simulink library "foc_blocks"  (R2020b)
settings: Solver=ode45  StartTime=0.0  StopTime=10.0  RelTol=1e-3  EnableMultiTasking=on
values from neighbouring files (symbols this model uses):
  ClockFrequency = 100    [setup_DF_fixp16_alu_av.m]    (also in setup_sim_DF_fixp16_alu.m; setup_verify_DF_fixp16_alu.m)
  constfractionlengthIn = 10    [setup_DF_fixp16_alu_av.m]    (also in setup_sim_DF_fixp16_alu.m; setup_verify_DF_fixp16_alu.m)
  constwordlengthIn = 16    [setup_DF_fixp16_alu_av.m]    (also in setup_sim_DF_fixp16_alu.m; setup_verify_DF_fixp16_alu.m)
  DSPBASampleTime = FoldingFactor / (ClockFrequency * 1e6)    (= 5e-06)    [setup_DF_fixp16_alu_av.m]    (also in setup_sim_DF_fixp16_alu.m; setup_verify_DF_fixp16_alu.m)
  FoldingFactor = 500    [setup_DF_fixp16_alu_av.m]    (also in setup_sim_DF_fixp16_alu.m; setup_verify_DF_fixp16_alu.m)
undefined symbols (not defined in the file or in its folder): AdvDSPBChannelOutDisplay, dpoly, dspba_ChannelInVis, dspba_ChannelOutVis, dspba_internal_get_channel_ports, evalAionMaskParam, latency, primtype, value, x
libraries: DSPBAPrim x559, AlteraGenericMotorLibrary x20, $bdroot x9, DSPBAUtilities x4, DSPBAControl x4
(part 4 of 6)

== system foc_blocks/FL_float_filt/FP_CP1_DSPBA1 ==
  note: Park & Clarke Transform
  I_uw : Inport
  cos_phi_el : Inport  Port=2
  sin_phi_el : Inport  Port=3
  Add : DSPBAPrim/Add  primtype=add  nInputs=evalAionMaskParam(gcb,'value',1)  nOutputs=1  omode=Inherit via internal rule  otype=sfix(16)  scale=2^-15  rndmethod=Unbiased  factor=1  satmethod=Symmetric  shift_vec=[0 1 2 -1]  value=2  inPortNames=[' '; ' ';]  outPortNames=[' ']  dspbaimage=dspba_prim.jpg  text=fprintf('+');  style=Optimised  visibilities=1032  genFPC=off  floatRounding=faithful  advOptions=[]  version=20130821
  Add1 : DSPBAPrim/Add  primtype=add  nInputs=evalAionMaskParam(gcb,'value',1)  nOutputs=1  omode=Inherit via internal rule with word growth  otype=sfix(16)  scale=2^-15  rndmethod=Unbiased  factor=1  satmethod=Symmetric  shift_vec=[0 1 2 -1]  value=2  inPortNames=[' '; ' ';]  outPortNames=[' ']  dspbaimage=dspba_prim.jpg  text=fprintf('+');  style=Optimised  visibilities=1032  genFPC=off  floatRounding=faithful  advOptions=[]  version=20130821
  Altera DSP Builder Advanced : AlteraGenericMotorLibrary/FP_Cur_Ctrl_DSPBA/Altera DSP Builder Advanced  SystemSampleTime=-1  VariantActivationTime=update diagram  Latency=0  AutoFrameSizeCalculation=off
  Demux1 : Demux  Outputs=2
  FPGain : Subsystem  mask{constVal=2}
      mask prompts: constVal "Gain"
      mask Display: color('w');fprintf('FP Gain\n%s', num2str(constVal));port_label('input',1,'a');port_label('output',1,'q');
  FPGain1 : Subsystem  mask{constVal=-1/sqrt(3)}
      mask prompts: constVal "Gain"
      mask Display: color('w');fprintf('FP Gain\n%s', num2str(constVal));port_label('input',1,'a');port_label('output',1,'q');
  Mult{,1..3} (4 alike) : DSPBAPrim/Mult  primtype=mult  nInputs=2  nOutputs=1  omode=Inherit via internal rule  otype=sfix(16)  scale=2^-15  rndmethod=Unbiased  factor=1  satmethod=Symmetric  shift_vec=[0 1 2 -1]  value=0  inPortNames=[' '; ' ';]  outPortNames=[' ']  dspbaimage=dspba_prim.jpg  text=fprintf('X');  style=Optimised  visibilities=8  floatPrecision=float32_m23  floatRounding=faithful  advOptions=[]  version=20130115
  Mux1 : Mux  Inputs=2
  Sub1 : DSPBAPrim/Sub  primtype=sub  nInputs=2  nOutputs=1  omode=Inherit via internal rule  otype=sfix(16)  scale=2^-15  rndmethod=Unbiased  factor=1  satmethod=Symmetric  shift_vec=[0 1 2 -1]  value=0  inPortNames=['+'; '-';]  outPortNames=[' ']  dspbaimage=dspba_prim.jpg  text=fprintf('-');  style=Optimised  visibilities=8  floatRounding=faithful  advOptions=[]  version=20130115
  I_dq : Outport
  wires:
  Sub1/1 -> Mux1/2
  Add/1 -> Mux1/1
  Mux1/1 -> I_dq/1
  Mult3/1 -> Sub1/1
  Mult2/1 -> Sub1/2
  Mult1/1 -> Add/2
  Mult/1 -> Add/1
  cos_phi_el/1 -> Mult/2, Mult3/2
  FPGain1/1(Out1) -> Mult1/1, Mult3/1
  Demux1/1 -> Mult/1, Mult2/2, Add1/1
  Demux1/2 -> FPGain/1(In1)
  I_uw/1 -> Demux1/1
  sin_phi_el/1 -> Mult1/2, Mult2/1
  Add1/1 -> FPGain1/1(In1)
  FPGain/1(Out1) -> Add1/2

== system foc_blocks/FL_float_filt/FP_Inv_Park1 ==
  note: Inverse Park Transform
  I_dq : Inport
  cos_phi_el : Inport  Port=2
  sin_phi_el : Inport  Port=3
  Add : DSPBAPrim/Add  primtype=add  nInputs=evalAionMaskParam(gcb,'value',1)  nOutputs=1  omode=Inherit via internal rule  otype=sfix(16)  scale=2^-15  rndmethod=Unbiased  factor=1  satmethod=Symmetric  shift_vec=[0 1 2 -1]  value=2  inPortNames=[' '; ' ';]  outPortNames=[' ']  dspbaimage=dspba_prim.jpg  text=fprintf('+');  style=Optimised  visibilities=1032  genFPC=off  floatRounding=faithful  advOptions=[]  version=20130821
  Altera DSP Builder Advanced : AlteraGenericMotorLibrary/FP_Cur_Ctrl_DSPBA/Altera DSP Builder Advanced  SystemSampleTime=-1  VariantActivationTime=update diagram  Latency=0  AutoFrameSizeCalculation=off
  Demux1 : Demux  Outputs=2
  Mult{1..4} (4 alike) : DSPBAPrim/Mult  primtype=mult  nInputs=2  nOutputs=1  omode=Inherit via internal rule  otype=sfix(16)  scale=2^-15  rndmethod=Unbiased  factor=1  satmethod=Symmetric  shift_vec=[0 1 2 -1]  value=0  inPortNames=[' '; ' ';]  outPortNames=[' ']  dspbaimage=dspba_prim.jpg  text=fprintf('X');  style=Optimised  visibilities=8  floatPrecision=float32_m23  floatRounding=faithful  advOptions=[]  version=20130115
  Mux2 : Mux  Inputs=2
  Sub1 : DSPBAPrim/Sub  primtype=sub  nInputs=2  nOutputs=1  omode=Inherit via internal rule  otype=sfix(16)  scale=2^-15  rndmethod=Unbiased  factor=1  satmethod=Symmetric  shift_vec=[0 1 2 -1]  value=0  inPortNames=['+'; '-';]  outPortNames=[' ']  dspbaimage=dspba_prim.jpg  text=fprintf('-');  style=Optimised  visibilities=8  floatRounding=faithful  advOptions=[]  version=20130115
  I_alpha_beta : Outport
  wires:
  Mult2/1 -> Add/1
  Mult1/1 -> Add/2
  Mult4/1 -> Sub1/1
  Mult3/1 -> Sub1/2
  Demux1/1 -> Mult2/1, Mult4/1  "I_d"
  cos_phi_el/1 -> Mult1/2, Mult4/2
  Demux1/2 -> Mult1/1, Mult3/1  "I_q"
  sin_phi_el/1 -> Mult2/2, Mult3/2
  I_dq/1 -> Demux1/1
  Mux2/1 -> I_alpha_beta/1
  Sub1/1 -> Mux2/1
  Add/1 -> Mux2/2

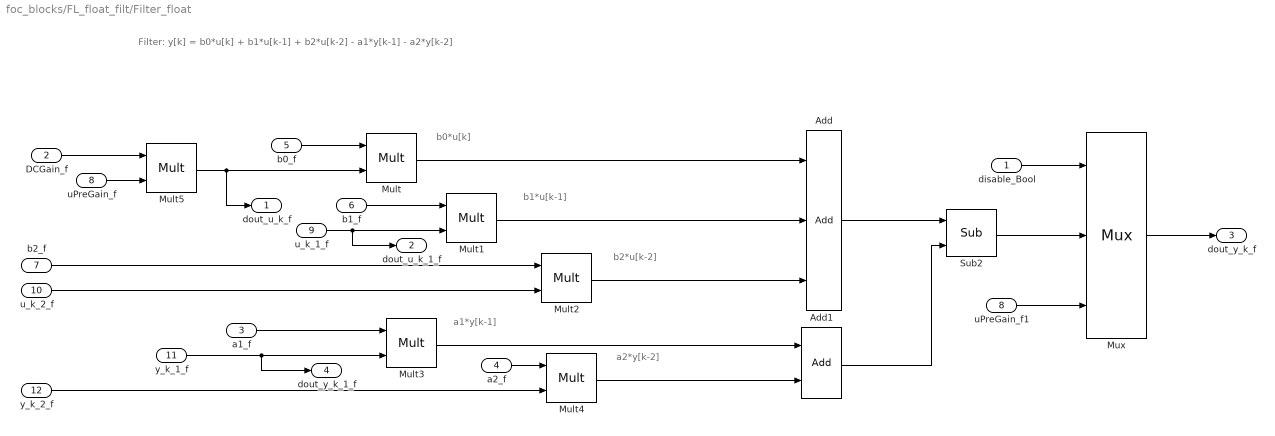
== system foc_blocks/FL_float_filt/Filter_float ==
  note: b0*u[k]
  note: b1*u[k-1]
  note: b2*u[k-2]
  note: a1*y[k-1]
  note: a2*y[k-2]
  note: Filter: y[k] = b0*u[k] + b1*u[k-1] + b2*u[k-2] - a1*y[k-1] - a2*y[k-2]
  disable_Bool : Inport
  DCGain_f : Inport  Port=2
  a1_f : Inport  Port=3
  a2_f : Inport  Port=4
  b0_f : Inport  Port=5
  b1_f : Inport  Port=6
  b2_f : Inport  Port=7
  uPreGain_f : Inport  Port=8
  u_k_1_f : Inport  Port=9
  u_k_2_f : Inport  Port=10
  y_k_1_f : Inport  Port=11
  y_k_2_f : Inport  Port=12
  Add : DSPBAPrim/Add  primtype=add  nInputs=evalAionMaskParam(gcb,'value',1)  nOutputs=1  omode=Inherit via internal rule  otype=sfix(16)  scale=2^-15  rndmethod=Unbiased  factor=1  satmethod=Symmetric  shift_vec=[0 1 2 -1]  value=3  inPortNames=[' '; ' ';]  outPortNames=[' ']  dspbaimage=dspba_prim.jpg  text=fprintf('+');  style=Optimised  visibilities=1032  genFPC=off  floatRounding=faithful  advOptions=[]  version=20130821
  Add1 : DSPBAPrim/Add  primtype=add  nInputs=evalAionMaskParam(gcb,'value',1)  nOutputs=1  omode=Inherit via internal rule  otype=sfix(16)  scale=2^-15  rndmethod=Unbiased  factor=1  satmethod=Symmetric  shift_vec=[0 1 2 -1]  value=2  inPortNames=[' '; ' ';]  outPortNames=[' ']  dspbaimage=dspba_prim.jpg  text=fprintf('+');  style=Optimised  visibilities=1032  genFPC=off  floatRounding=faithful  advOptions=[]  version=20130821
  Mult{,1..5} (6 alike) : DSPBAPrim/Mult  primtype=mult  nInputs=2  nOutputs=1  omode=Inherit via internal rule  otype=sfix(16)  scale=2^-15  rndmethod=Unbiased  factor=1  satmethod=Symmetric  shift_vec=[0 1 2 -1]  value=0  inPortNames=[' '; ' ';]  outPortNames=[' ']  dspbaimage=dspba_prim.jpg  text=fprintf('X');  style=Optimised  visibilities=8  floatPrecision=float32_m23  floatRounding=faithful  advOptions=[]  version=20130115
  Mux : DSPBAPrim/Mux  primtype=mux  nInputs=evalAionMaskParam(gcb,'value',1)+1  nOutputs=1  omode=Inherit via internal rule  otype=sfix(16)  scale=2^-15  rndmethod=Unbiased  factor=1  satmethod=Symmetric  shift_vec=[0 1 2 -1]  value=2  inPortNames=['s'; 'd0'; 'd1'; 'd2'; 'd3'; 'd4'; 'd5'; 'd6'; 'd7'; 'd8'; 'd9';]  outPortNames=[' ']  dspbaimage=dspba_prim.jpg  text=fprintf('%s', primtype);  style=Optimised  visibilities=1032  version=20131025
  Sub2 : DSPBAPrim/Sub  primtype=sub  nInputs=2  nOutputs=1  omode=Inherit via internal rule  otype=sfix(16)  scale=2^-15  rndmethod=Unbiased  factor=1  satmethod=Symmetric  shift_vec=[0 1 2 -1]  value=0  inPortNames=['+'; '-';]  outPortNames=[' ']  dspbaimage=dspba_prim.jpg  text=fprintf('-');  style=Optimised  visibilities=8  floatRounding=faithful  advOptions=[]  version=20130115
  uPreGain_f1 : InportShadow  Port=8
  dout_u_k_f : Outport
  dout_u_k_1_f : Outport  Port=2
  dout_y_k_f : Outport  Port=3
  dout_y_k_1_f : Outport  Port=4
  wires:
  b1_f/1 -> Mult1/1
  y_k_1_f/1 -> dout_y_k_1_f/1, Mult3/2
  u_k_1_f/1 -> dout_u_k_1_f/1, Mult1/2
  Mult4/1 -> Add1/2
  b0_f/1 -> Mult/1
  a1_f/1 -> Mult3/1
  u_k_2_f/1 -> Mult2/2
  b2_f/1 -> Mult2/1
  Mult3/1 -> Add1/1
  Add1/1 -> Sub2/2
  Add/1 -> Sub2/1
  Mult1/1 -> Add/2
  Mult/1 -> Add/1
  a2_f/1 -> Mult4/1
  Mult2/1 -> Add/3
  y_k_2_f/1 -> Mult4/2
  Mult5/1 -> dout_u_k_f/1, Mult/2
  DCGain_f/1 -> Mult5/1
  uPreGain_f/1 -> Mult5/2
  disable_Bool/1 -> Mux/1
  uPreGain_f1/1 -> Mux/3
  Sub2/1 -> Mux/2
  Mux/1 -> dout_y_k_f/1

== system foc_blocks/FL_float_filt/Filter_float1 ==
  note: Filter: y[k] = b0*u[k] + b1*u[k-1] + b2*u[k-2] - a1*y[k-1] - a2*y[k-2]
  note: a2*y[k-2]
  note: a1*y[k-1]
  note: b2*u[k-2]
  note: b1*u[k-1]
  note: b0*u[k]
  disable_Bool : Inport
  DCGain_f : Inport  Port=2
  a1_f : Inport  Port=3
  a2_f : Inport  Port=4
  b0_f : Inport  Port=5
  b1_f : Inport  Port=6
  b2_f : Inport  Port=7
  uPreGain_f : Inport  Port=8
  u_k_1_f : Inport  Port=9
  u_k_2_f : Inport  Port=10
  y_k_1_f : Inport  Port=11
  y_k_2_f : Inport  Port=12
  Add : DSPBAPrim/Add  primtype=add  nInputs=evalAionMaskParam(gcb,'value',1)  nOutputs=1  omode=Inherit via internal rule  otype=sfix(16)  scale=2^-15  rndmethod=Unbiased  factor=1  satmethod=Symmetric  shift_vec=[0 1 2 -1]  value=3  inPortNames=[' '; ' ';]  outPortNames=[' ']  dspbaimage=dspba_prim.jpg  text=fprintf('+');  style=Optimised  visibilities=1032  genFPC=off  floatRounding=faithful  advOptions=[]  version=20130821
  Add1 : DSPBAPrim/Add  primtype=add  nInputs=evalAionMaskParam(gcb,'value',1)  nOutputs=1  omode=Inherit via internal rule  otype=sfix(16)  scale=2^-15  rndmethod=Unbiased  factor=1  satmethod=Symmetric  shift_vec=[0 1 2 -1]  value=2  inPortNames=[' '; ' ';]  outPortNames=[' ']  dspbaimage=dspba_prim.jpg  text=fprintf('+');  style=Optimised  visibilities=1032  genFPC=off  floatRounding=faithful  advOptions=[]  version=20130821
  Mult{,1..5} (6 alike) : DSPBAPrim/Mult  primtype=mult  nInputs=2  nOutputs=1  omode=Inherit via internal rule  otype=sfix(16)  scale=2^-15  rndmethod=Unbiased  factor=1  satmethod=Symmetric  shift_vec=[0 1 2 -1]  value=0  inPortNames=[' '; ' ';]  outPortNames=[' ']  dspbaimage=dspba_prim.jpg  text=fprintf('X');  style=Optimised  visibilities=8  floatPrecision=float32_m23  floatRounding=faithful  advOptions=[]  version=20130115
  Mux : DSPBAPrim/Mux  primtype=mux  nInputs=evalAionMaskParam(gcb,'value',1)+1  nOutputs=1  omode=Inherit via internal rule  otype=sfix(16)  scale=2^-15  rndmethod=Unbiased  factor=1  satmethod=Symmetric  shift_vec=[0 1 2 -1]  value=2  inPortNames=['s'; 'd0'; 'd1'; 'd2'; 'd3'; 'd4'; 'd5'; 'd6'; 'd7'; 'd8'; 'd9';]  outPortNames=[' ']  dspbaimage=dspba_prim.jpg  text=fprintf('%s', primtype);  style=Optimised  visibilities=1032  version=20131025
  Sub2 : DSPBAPrim/Sub  primtype=sub  nInputs=2  nOutputs=1  omode=Inherit via internal rule  otype=sfix(16)  scale=2^-15  rndmethod=Unbiased  factor=1  satmethod=Symmetric  shift_vec=[0 1 2 -1]  value=0  inPortNames=['+'; '-';]  outPortNames=[' ']  dspbaimage=dspba_prim.jpg  text=fprintf('-');  style=Optimised  visibilities=8  floatRounding=correct  advOptions=[]  version=20130115
  uPreGain_f1 : InportShadow  Port=8
  dout_u_k_f : Outport
  dout_u_k_1_f : Outport  Port=2
  dout_y_k_f : Outport  Port=3
  dout_y_k_1_f : Outport  Port=4
  wires:
  Mux/1 -> dout_y_k_f/1
  Sub2/1 -> Mux/2
  uPreGain_f1/1 -> Mux/3
  disable_Bool/1 -> Mux/1
  uPreGain_f/1 -> Mult5/2
  DCGain_f/1 -> Mult5/1
  Mult5/1 -> Mult/2, dout_u_k_f/1
  y_k_2_f/1 -> Mult4/2
  Mult2/1 -> Add/3
  a2_f/1 -> Mult4/1
  Mult/1 -> Add/1
  Mult1/1 -> Add/2
  Add/1 -> Sub2/1
  Add1/1 -> Sub2/2
  Mult3/1 -> Add1/1
  b2_f/1 -> Mult2/1
  u_k_2_f/1 -> Mult2/2
  a1_f/1 -> Mult3/1
  b0_f/1 -> Mult/1
  Mult4/1 -> Add1/2
  u_k_1_f/1 -> Mult1/2, dout_u_k_1_f/1
  y_k_1_f/1 -> Mult3/2, dout_y_k_1_f/1
  b1_f/1 -> Mult1/1

== system foc_blocks/FL_float_filt/PI_Ctrl_D_DSPBA ==
  note: Simple Proportional + Integral (PI) Controller
  note: Error Input
  note: Proportional Gain
  note: Integral Gain
  note: Saturate
  note: Saturate
  note: Correction Output
  note: Integral Output
  note: Integral Input
  note: Saturation limit
  PI_in : Inport
  Integral_in : Inport  Port=2
  Kp_in : Inport  Port=3
  Ki_in : Inport  Port=4
  Add1 : DSPBAPrim/Add  primtype=add  nInputs=evalAionMaskParam(gcb,'value',1)  nOutputs=1  omode=Inherit via internal rule with word growth  otype=sfix(16)  scale=2^-15  rndmethod=Unbiased  factor=1  satmethod=Symmetric  shift_vec=[0 1 2 -1]  value=2  inPortNames=[' '; ' ';]  outPortNames=[' ']  dspbaimage=dspba_prim.jpg  text=fprintf('+');  style=Optimised  visibilities=1032  genFPC=off  floatRounding=faithful  advOptions=[]  version=20130821
  Add4 : DSPBAPrim/Add  primtype=add  nInputs=evalAionMaskParam(gcb,'value',1)  nOutputs=1  omode=Inherit via internal rule with word growth  otype=sfix(16)  scale=2^-15  rndmethod=Unbiased  factor=1  satmethod=Symmetric  shift_vec=[0 1 2 -1]  value=2  inPortNames=[' '; ' ';]  outPortNames=[' ']  dspbaimage=dspba_prim.jpg  text=fprintf('+');  style=Optimised  visibilities=1032  genFPC=off  floatRounding=faithful  advOptions=[]  version=20130821
  Altera DSP Builder Advanced : AlteraGenericMotorLibrary/FP_Cur_Ctrl_DSPBA/Altera DSP Builder Advanced  SystemSampleTime=-1  VariantActivationTime=update diagram  Latency=0  AutoFrameSizeCalculation=off
  FPSaturate1 : Subsystem
      mask Display: color('w');fprintf('FP Var Sat\n');port_label('input',1,'a');port_label('input',2,'limit');port_label('output',1,'q');
  FPSaturate2 : Subsystem
      mask Display: color('w');fprintf('FP Var Sat\n');port_label('input',1,'a');port_label('input',2,'limit');port_label('output',1,'q');
  Limit : DSPBAPrim/Const  primtype=const  nInputs=0  nOutputs=1  omode=Specify via dialog  otype=fpDT  scale=1  rndmethod=Unbiased  factor=1  satmethod=Symmetric  shift_vec=[0 1 2 -1]  value=0.95*2^(constwordlengthIn-constfractionlengthIn-1)  inPortNames=['+'; '+';]  outPortNames=[' ']  dspbaimage=dspba_prim.jpg  text=fprintf('%s', num2str(value));  style=Optimised  visibilities=8 + 1024  floatPrecision=float32_m23  version=20120820
  Mult1 : DSPBAPrim/Mult  primtype=mult  nInputs=2  nOutputs=1  omode=Inherit via internal rule  otype=sfix(16)  scale=2^-15  rndmethod=Unbiased  factor=1  satmethod=Symmetric  shift_vec=[0 1 2 -1]  value=0  inPortNames=[' '; ' ';]  outPortNames=[' ']  dspbaimage=dspba_prim.jpg  text=fprintf('X');  style=Optimised  visibilities=8  floatPrecision=float32_m23  floatRounding=faithful  advOptions=[]  version=20130115
  Mult4 : DSPBAPrim/Mult  primtype=mult  nInputs=2  nOutputs=1  omode=Inherit via internal rule  otype=sfix(16)  scale=2^-15  rndmethod=Unbiased  factor=1  satmethod=Symmetric  shift_vec=[0 1 2 -1]  value=0  inPortNames=[' '; ' ';]  outPortNames=[' ']  dspbaimage=dspba_prim.jpg  text=fprintf('X');  style=Optimised  visibilities=8  floatPrecision=float32_m23  floatRounding=faithful  advOptions=[]  version=20130115
  PI_out : Outport
  I_out : Outport  Port=2
  wires:
  FPSaturate1/1(q) -> PI_out/1
  Add1/1 -> FPSaturate1/1(a)
  PI_in/1 -> Mult4/1, Mult1/1
  Mult4/1 -> Add1/1
  FPSaturate2/1(q) -> Add1/2, I_out/1
  Add4/1 -> FPSaturate2/1(a)
  Integral_in/1 -> Add4/2
  Kp_in/1 -> Mult4/2
  Mult1/1 -> Add4/1
  Ki_in/1 -> Mult1/2
  Limit/1 -> FPSaturate1/2(limit), FPSaturate2/2(limit)

== system foc_blocks/FL_float_filt/PI_Ctrl_D_DSPBA1 ==
  note: Integral Input
  note: Integral Output
  note: Correction Output
  note: Saturate
  note: Saturate
  note: Integral Gain
  note: Proportional Gain
  note: Error Input
  note: Simple Proportional + Integral (PI) Controller
  note: Saturation limit
  PI_in : Inport
  Integral_in : Inport  Port=2
  Kp_in : Inport  Port=3
  Ki_in : Inport  Port=4
  Add1 : DSPBAPrim/Add  primtype=add  nInputs=evalAionMaskParam(gcb,'value',1)  nOutputs=1  omode=Inherit via internal rule with word growth  otype=sfix(16)  scale=2^-15  rndmethod=Unbiased  factor=1  satmethod=Symmetric  shift_vec=[0 1 2 -1]  value=2  inPortNames=[' '; ' ';]  outPortNames=[' ']  dspbaimage=dspba_prim.jpg  text=fprintf('+');  style=Optimised  visibilities=1032  genFPC=off  floatRounding=faithful  advOptions=[]  version=20130821
  Add4 : DSPBAPrim/Add  primtype=add  nInputs=evalAionMaskParam(gcb,'value',1)  nOutputs=1  omode=Inherit via internal rule with word growth  otype=sfix(16)  scale=2^-15  rndmethod=Unbiased  factor=1  satmethod=Symmetric  shift_vec=[0 1 2 -1]  value=2  inPortNames=[' '; ' ';]  outPortNames=[' ']  dspbaimage=dspba_prim.jpg  text=fprintf('+');  style=Optimised  visibilities=1032  genFPC=off  floatRounding=faithful  advOptions=[]  version=20130821
  Altera DSP Builder Advanced : AlteraGenericMotorLibrary/FP_Cur_Ctrl_DSPBA/Altera DSP Builder Advanced  SystemSampleTime=-1  VariantActivationTime=update diagram  Latency=0  AutoFrameSizeCalculation=off
  FPSaturate1 : Subsystem
      mask Display: color('w');fprintf('FP Var Sat\n');port_label('input',1,'a');port_label('input',2,'limit');port_label('output',1,'q');
  FPSaturate2 : Subsystem
      mask Display: color('w');fprintf('FP Var Sat\n');port_label('input',1,'a');port_label('input',2,'limit');port_label('output',1,'q');
  Limit : DSPBAPrim/Const  primtype=const  nInputs=0  nOutputs=1  omode=Specify via dialog  otype=fpDT  scale=1  rndmethod=Unbiased  factor=1  satmethod=Symmetric  shift_vec=[0 1 2 -1]  value=0.95*2^(constwordlengthIn-constfractionlengthIn-1)  inPortNames=['+'; '+';]  outPortNames=[' ']  dspbaimage=dspba_prim.jpg  text=fprintf('%s', num2str(value));  style=Optimised  visibilities=8 + 1024  floatPrecision=float32_m23  version=20120820
  Mult1 : DSPBAPrim/Mult  primtype=mult  nInputs=2  nOutputs=1  omode=Inherit via internal rule  otype=sfix(16)  scale=2^-15  rndmethod=Unbiased  factor=1  satmethod=Symmetric  shift_vec=[0 1 2 -1]  value=0  inPortNames=[' '; ' ';]  outPortNames=[' ']  dspbaimage=dspba_prim.jpg  text=fprintf('X');  style=Optimised  visibilities=8  floatPrecision=float32_m23  floatRounding=faithful  advOptions=[]  version=20130115
  Mult4 : DSPBAPrim/Mult  primtype=mult  nInputs=2  nOutputs=1  omode=Inherit via internal rule  otype=sfix(16)  scale=2^-15  rndmethod=Unbiased  factor=1  satmethod=Symmetric  shift_vec=[0 1 2 -1]  value=0  inPortNames=[' '; ' ';]  outPortNames=[' ']  dspbaimage=dspba_prim.jpg  text=fprintf('X');  style=Optimised  visibilities=8  floatPrecision=float32_m23  floatRounding=faithful  advOptions=[]  version=20130115
  PI_out : Outport
  I_out : Outport  Port=2
  wires:
  Ki_in/1 -> Mult1/2
  Mult1/1 -> Add4/1
  Kp_in/1 -> Mult4/2
  Integral_in/1 -> Add4/2
  Add4/1 -> FPSaturate2/1(a)
  FPSaturate2/1(q) -> I_out/1, Add1/2
  Mult4/1 -> Add1/1
  PI_in/1 -> Mult1/1, Mult4/1
  Add1/1 -> FPSaturate1/1(a)
  FPSaturate1/1(q) -> PI_out/1
  Limit/1 -> FPSaturate2/2(limit), FPSaturate1/2(limit)

== system foc_blocks/FilterLatches/latches ==
  In_u_k_f : Inport
  In_u_k_1_f : Inport  Port=2
  In_y_k_f : Inport  Port=3
  In_y_k_1_f : Inport  Port=4
  valid_in : Inport  Port=5
  reset_flag_Bool : Inport  Port=6
  reset_value_u_k_f : Inport  Port=7
  Latch_u_k_1 : Subsystem
  Latch_u_k_2 : $bdroot/FilterLatches/latches/Latch_u_k_1  SystemSampleTime=-1  VariantActivationTime=update diagram  Latency=0  AutoFrameSizeCalculation=off
  Latch_u_k_3 : $bdroot/FilterLatches/latches/Latch_u_k_1  SystemSampleTime=-1  VariantActivationTime=update diagram  Latency=0  AutoFrameSizeCalculation=off
  Latch_u_k_4 : $bdroot/FilterLatches/latches/Latch_u_k_1  SystemSampleTime=-1  VariantActivationTime=update diagram  Latency=0  AutoFrameSizeCalculation=off
  Out_u_k_1_f : Outport
  Out_u_k_2_f : Outport  Port=2
  Out_y_k_1_f : Outport  Port=3
  Out_y_k_2_f : Outport  Port=4
  wires:
  reset_flag_Bool/1 -> Latch_u_k_2/3, Latch_u_k_4/3, Latch_u_k_3/3, Latch_u_k_1/3(load)
  valid_in/1 -> Latch_u_k_2/2, Latch_u_k_4/2, Latch_u_k_3/2, Latch_u_k_1/2(valid_in)
  reset_value_u_k_f/1 -> Latch_u_k_2/4, Latch_u_k_4/4, Latch_u_k_3/4, Latch_u_k_1/4(load_value)
  In_u_k_f/1 -> Latch_u_k_1/1(data_in)
  Latch_u_k_1/1(data_out) -> Out_u_k_1_f/1
  In_u_k_1_f/1 -> Latch_u_k_2/1
  Latch_u_k_2/1 -> Out_u_k_2_f/1
  Latch_u_k_4/1 -> Out_y_k_2_f/1
  In_y_k_f/1 -> Latch_u_k_3/1
  In_y_k_1_f/1 -> Latch_u_k_4/1
  Latch_u_k_3/1 -> Out_y_k_1_f/1

== system foc_blocks/fb_latches/latches ==
  din1 : Inport
  valid_in : Inport  Port=2
  din2 : Inport  Port=3
  load : Inport  Port=4
  RL : Subsystem
  RL1 : Subsystem
  SameDT2 : DSPBAControl/SameDT
  reset_integ2 : DSPBAPrim/Const  primtype=const  nInputs=0  nOutputs=1  omode=Inherit via back propagation  otype=fpDT  scale=1  rndmethod=Unbiased  factor=1  satmethod=Symmetric  shift_vec=[0 1 2 -1]  value=0  inPortNames=['+'; '+';]  outPortNames=[' ']  dspbaimage=dspba_prim.jpg  text=fprintf('%s', num2str(value));  style=Optimised  visibilities=8 + 1024  floatPrecision=float32_m23  version=20120820
  Out1 : Outport
  Out2 : Outport  Port=2
  wires:
  RL1/1(data_out) -> Out2/1
  din2/1 -> SameDT2/1, RL1/1(data_in)
  RL/1(data_out) -> Out1/1
  din1/1 -> RL/1(data_in)
  reset_integ2/1 -> RL/4(load_value), SameDT2/2, RL1/4(load_value)
  valid_in/1 -> RL/2(valid_in), RL1/2(valid_in)
  load/1 -> RL/3(load), RL1/3(load)

== system foc_blocks/FL_fixp16/FP_CP1_DSPBA/FixedGain ==
  In1 : Inport
  Const : DSPBAPrim/Const  primtype=const  nInputs=0  nOutputs=1  omode=Specify via dialog  otype=constOTypeIn  scale=constScaleIn  rndmethod=Unbiased  factor=1  satmethod=Symmetric  shift_vec=[0 1 2 -1]  value=constVal  inPortNames=['+'; '+';]  outPortNames=[' ']  dspbaimage=dspba_prim.jpg  text=fprintf('%s', num2str(value));  style=Optimised  visibilities=8 + 1024  floatPrecision=float32_m23  version=20120820
  Mult : DSPBAPrim/Mult  primtype=mult  nInputs=2  nOutputs=1  omode=Specify via dialog  otype=constOTypeIn  scale=constScaleIn  rndmethod=Unbiased  factor=1  satmethod=Symmetric  shift_vec=[0 1 2 -1]  value=0  inPortNames=[' '; ' ';]  outPortNames=[' ']  dspbaimage=dspba_prim.jpg  text=fprintf('X');  style=Optimised  visibilities=8  floatPrecision=float32_m23  floatRounding=correct  advOptions=[]  version=20130115
  Out1 : Outport
  wires:
  Const/1 -> Mult/2
  Mult/1 -> Out1/1
  In1/1 -> Mult/1

== system foc_blocks/FL_fixp16/FP_CP1_DSPBA/FixedGain1 ==
  In1 : Inport
  Const : DSPBAPrim/Const  primtype=const  nInputs=0  nOutputs=1  omode=Specify via dialog  otype=constOTypeIn  scale=constScaleIn  rndmethod=Unbiased  factor=1  satmethod=Symmetric  shift_vec=[0 1 2 -1]  value=constVal  inPortNames=['+'; '+';]  outPortNames=[' ']  dspbaimage=dspba_prim.jpg  text=fprintf('%s', num2str(value));  style=Optimised  visibilities=8 + 1024  floatPrecision=float32_m23  version=20120820
  Mult : DSPBAPrim/Mult  primtype=mult  nInputs=2  nOutputs=1  omode=Specify via dialog  otype=constOTypeIn  scale=constScaleIn  rndmethod=Unbiased  factor=1  satmethod=Symmetric  shift_vec=[0 1 2 -1]  value=0  inPortNames=[' '; ' ';]  outPortNames=[' ']  dspbaimage=dspba_prim.jpg  text=fprintf('X');  style=Optimised  visibilities=8  floatPrecision=float32_m23  floatRounding=correct  advOptions=[]  version=20130115
  Out1 : Outport
  wires:
  In1/1 -> Mult/1
  Mult/1 -> Out1/1
  Const/1 -> Mult/2

== system foc_blocks/FL_fixp16/PI_Ctrl_D_DSPBA/Fixed Saturate1 ==
  In1 : Inport
  limit : Inport  Port=2
  MinMax : DSPBAPrim/MinMax  primtype=minmaxfunc  nInputs=2  nOutputs=1  omode=Inherit via internal rule  otype=constOTypeIn  scale=constScaleIn  rndmethod=Unbiased  factor=1  satmethod=Symmetric  shift_vec=[0 1 2 -1]  value=0  inPortNames=[' '; ' ';]  outPortNames=[' ']  dspbaimage=dspba_prim.jpg  text=disp('min');  style=Optimised  visibilities=8+2^17  functionExpr=min  advOptions=[]  version=20121130
  MinMax1 : DSPBAPrim/MinMax  primtype=minmaxfunc  nInputs=2  nOutputs=1  omode=Specify via dialog  otype=constOTypeIn  scale=constScaleIn  rndmethod=Unbiased  factor=1  satmethod=Symmetric  shift_vec=[0 1 2 -1]  value=0  inPortNames=[' '; ' ';]  outPortNames=[' ']  dspbaimage=dspba_prim.jpg  text=disp('min');  style=Optimised  visibilities=8+2^17  functionExpr=max  advOptions=[]  version=20121130
  Sub : DSPBAPrim/Sub  primtype=sub  nInputs=2  nOutputs=1  omode=Inherit via internal rule  otype=sfix(16)  scale=2^-15  rndmethod=Unbiased  factor=1  satmethod=Symmetric  shift_vec=[0 1 2 -1]  value=0  inPortNames=['+'; '-';]  outPortNames=[' ']  dspbaimage=dspba_prim.jpg  text=fprintf('-');  style=Optimised  visibilities=8  floatRounding=correct  advOptions=[]  version=20130115
  const1 : DSPBAPrim/Const  primtype=const  nInputs=0  nOutputs=1  omode=Specify via dialog  otype=constOTypeIn  scale=constScaleIn  rndmethod=Unbiased  factor=1  satmethod=Symmetric  shift_vec=[0 1 2 -1]  value=0  inPortNames=['+'; '+';]  outPortNames=[' ']  dspbaimage=dspba_prim.jpg  text=fprintf('%s', num2str(value));  style=Optimised  visibilities=8 + 1024  floatPrecision=float32_m23  version=20120820
  Out1 : Outport
  wires:
  limit/1 -> MinMax/1, Sub/2
  const1/1 -> Sub/1
  In1/1 -> MinMax/2
  Sub/1 -> MinMax1/2
  MinMax1/1 -> Out1/1
  MinMax/1 -> MinMax1/1

== system foc_blocks/FL_fixp16/PI_Ctrl_D_DSPBA/Fixed Saturate2 ==
  In1 : Inport
  limit : Inport  Port=2
  MinMax : DSPBAPrim/MinMax  primtype=minmaxfunc  nInputs=2  nOutputs=1  omode=Inherit via internal rule  otype=constOTypeIn  scale=constScaleIn  rndmethod=Unbiased  factor=1  satmethod=Symmetric  shift_vec=[0 1 2 -1]  value=0  inPortNames=[' '; ' ';]  outPortNames=[' ']  dspbaimage=dspba_prim.jpg  text=disp('min');  style=Optimised  visibilities=8+2^17  functionExpr=min  advOptions=[]  version=20121130
  MinMax1 : DSPBAPrim/MinMax  primtype=minmaxfunc  nInputs=2  nOutputs=1  omode=Specify via dialog  otype=constOTypeIn  scale=constScaleIn  rndmethod=Unbiased  factor=1  satmethod=Symmetric  shift_vec=[0 1 2 -1]  value=0  inPortNames=[' '; ' ';]  outPortNames=[' ']  dspbaimage=dspba_prim.jpg  text=disp('min');  style=Optimised  visibilities=8+2^17  functionExpr=max  advOptions=[]  version=20121130
  Sub : DSPBAPrim/Sub  primtype=sub  nInputs=2  nOutputs=1  omode=Inherit via internal rule  otype=sfix(16)  scale=2^-15  rndmethod=Unbiased  factor=1  satmethod=Symmetric  shift_vec=[0 1 2 -1]  value=0  inPortNames=['+'; '-';]  outPortNames=[' ']  dspbaimage=dspba_prim.jpg  text=fprintf('-');  style=Optimised  visibilities=8  floatRounding=correct  advOptions=[]  version=20130115
  const1 : DSPBAPrim/Const  primtype=const  nInputs=0  nOutputs=1  omode=Specify via dialog  otype=constOTypeIn  scale=constScaleIn  rndmethod=Unbiased  factor=1  satmethod=Symmetric  shift_vec=[0 1 2 -1]  value=0  inPortNames=['+'; '+';]  outPortNames=[' ']  dspbaimage=dspba_prim.jpg  text=fprintf('%s', num2str(value));  style=Optimised  visibilities=8 + 1024  floatPrecision=float32_m23  version=20120820
  Out1 : Outport
  wires:
  limit/1 -> MinMax/1, Sub/2
  const1/1 -> Sub/1
  In1/1 -> MinMax/2
  Sub/1 -> MinMax1/2
  MinMax1/1 -> Out1/1
  MinMax/1 -> MinMax1/1

== system foc_blocks/FL_fixp16/PI_Ctrl_D_DSPBA1/Fixed Saturate1 ==
  In1 : Inport
  limit : Inport  Port=2
  MinMax : DSPBAPrim/MinMax  primtype=minmaxfunc  nInputs=2  nOutputs=1  omode=Inherit via internal rule  otype=constOTypeIn  scale=constScaleIn  rndmethod=Unbiased  factor=1  satmethod=Symmetric  shift_vec=[0 1 2 -1]  value=0  inPortNames=[' '; ' ';]  outPortNames=[' ']  dspbaimage=dspba_prim.jpg  text=disp('min');  style=Optimised  visibilities=8+2^17  functionExpr=min  advOptions=[]  version=20121130
  MinMax1 : DSPBAPrim/MinMax  primtype=minmaxfunc  nInputs=2  nOutputs=1  omode=Specify via dialog  otype=constOTypeIn  scale=constScaleIn  rndmethod=Unbiased  factor=1  satmethod=Symmetric  shift_vec=[0 1 2 -1]  value=0  inPortNames=[' '; ' ';]  outPortNames=[' ']  dspbaimage=dspba_prim.jpg  text=disp('min');  style=Optimised  visibilities=8+2^17  functionExpr=max  advOptions=[]  version=20121130
  Sub : DSPBAPrim/Sub  primtype=sub  nInputs=2  nOutputs=1  omode=Inherit via internal rule  otype=sfix(16)  scale=2^-15  rndmethod=Unbiased  factor=1  satmethod=Symmetric  shift_vec=[0 1 2 -1]  value=0  inPortNames=['+'; '-';]  outPortNames=[' ']  dspbaimage=dspba_prim.jpg  text=fprintf('-');  style=Optimised  visibilities=8  floatRounding=correct  advOptions=[]  version=20130115
  const1 : DSPBAPrim/Const  primtype=const  nInputs=0  nOutputs=1  omode=Specify via dialog  otype=constOTypeIn  scale=constScaleIn  rndmethod=Unbiased  factor=1  satmethod=Symmetric  shift_vec=[0 1 2 -1]  value=0  inPortNames=['+'; '+';]  outPortNames=[' ']  dspbaimage=dspba_prim.jpg  text=fprintf('%s', num2str(value));  style=Optimised  visibilities=8 + 1024  floatPrecision=float32_m23  version=20120820
  Out1 : Outport
  wires:
  MinMax/1 -> MinMax1/1
  MinMax1/1 -> Out1/1
  Sub/1 -> MinMax1/2
  In1/1 -> MinMax/2
  const1/1 -> Sub/1
  limit/1 -> Sub/2, MinMax/1

== system foc_blocks/FL_fixp16/PI_Ctrl_D_DSPBA1/Fixed Saturate2 ==
  In1 : Inport
  limit : Inport  Port=2
  MinMax : DSPBAPrim/MinMax  primtype=minmaxfunc  nInputs=2  nOutputs=1  omode=Inherit via internal rule  otype=constOTypeIn  scale=constScaleIn  rndmethod=Unbiased  factor=1  satmethod=Symmetric  shift_vec=[0 1 2 -1]  value=0  inPortNames=[' '; ' ';]  outPortNames=[' ']  dspbaimage=dspba_prim.jpg  text=disp('min');  style=Optimised  visibilities=8+2^17  functionExpr=min  advOptions=[]  version=20121130
  MinMax1 : DSPBAPrim/MinMax  primtype=minmaxfunc  nInputs=2  nOutputs=1  omode=Specify via dialog  otype=constOTypeIn  scale=constScaleIn  rndmethod=Unbiased  factor=1  satmethod=Symmetric  shift_vec=[0 1 2 -1]  value=0  inPortNames=[' '; ' ';]  outPortNames=[' ']  dspbaimage=dspba_prim.jpg  text=disp('min');  style=Optimised  visibilities=8+2^17  functionExpr=max  advOptions=[]  version=20121130
  Sub : DSPBAPrim/Sub  primtype=sub  nInputs=2  nOutputs=1  omode=Inherit via internal rule  otype=sfix(16)  scale=2^-15  rndmethod=Unbiased  factor=1  satmethod=Symmetric  shift_vec=[0 1 2 -1]  value=0  inPortNames=['+'; '-';]  outPortNames=[' ']  dspbaimage=dspba_prim.jpg  text=fprintf('-');  style=Optimised  visibilities=8  floatRounding=correct  advOptions=[]  version=20130115
  const1 : DSPBAPrim/Const  primtype=const  nInputs=0  nOutputs=1  omode=Specify via dialog  otype=constOTypeIn  scale=constScaleIn  rndmethod=Unbiased  factor=1  satmethod=Symmetric  shift_vec=[0 1 2 -1]  value=0  inPortNames=['+'; '+';]  outPortNames=[' ']  dspbaimage=dspba_prim.jpg  text=fprintf('%s', num2str(value));  style=Optimised  visibilities=8 + 1024  floatPrecision=float32_m23  version=20120820
  Out1 : Outport
  wires:
  MinMax/1 -> MinMax1/1
  MinMax1/1 -> Out1/1
  Sub/1 -> MinMax1/2
  In1/1 -> MinMax/2
  const1/1 -> Sub/1
  limit/1 -> Sub/2, MinMax/1

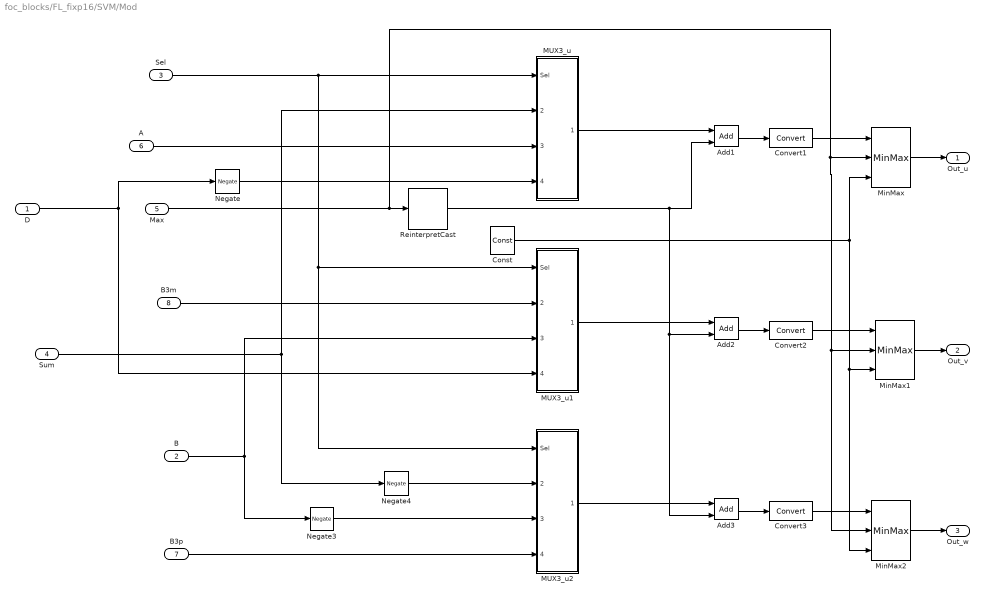
== system foc_blocks/FL_fixp16/SVM/Mod ==
  D : Inport
  B : Inport  Port=2
  Sel : Inport  Port=3
  Sum : Inport  Port=4
  Max : Inport  Port=5
  A : Inport  Port=6
  B3p : Inport  Port=7
  B3m : Inport  Port=8
  Add1 : DSPBAPrim/Add  primtype=add  nInputs=evalAionMaskParam(gcb,'value',1)  nOutputs=1  omode=Inherit via internal rule with word growth  otype=sfix(16)  scale=2^-15  rndmethod=Unbiased  factor=1  satmethod=Symmetric  shift_vec=[0 1 2 -1]  value=2  inPortNames=[' '; ' ';]  outPortNames=[' ']  dspbaimage=dspba_prim.jpg  text=fprintf('+');  style=Optimised  visibilities=1032+2^17+2^18+2^19  genFPC=off  floatRounding=correct  advOptions=[]  version=20130821
  Add2 : DSPBAPrim/Add  primtype=add  nInputs=evalAionMaskParam(gcb,'value',1)  nOutputs=1  omode=Inherit via internal rule with word growth  otype=sfix(16)  scale=2^-15  rndmethod=Unbiased  factor=1  satmethod=Symmetric  shift_vec=[0 1 2 -1]  value=2  inPortNames=[' '; ' ';]  outPortNames=[' ']  dspbaimage=dspba_prim.jpg  text=fprintf('+');  style=Optimised  visibilities=1032+2^17+2^18+2^19  genFPC=off  floatRounding=correct  advOptions=[]  version=20130821
  Add3 : DSPBAPrim/Add  primtype=add  nInputs=evalAionMaskParam(gcb,'value',1)  nOutputs=1  omode=Inherit via internal rule with word growth  otype=sfix(16)  scale=2^-15  rndmethod=Unbiased  factor=1  satmethod=Symmetric  shift_vec=[0 1 2 -1]  value=2  inPortNames=[' '; ' ';]  outPortNames=[' ']  dspbaimage=dspba_prim.jpg  text=fprintf('+');  style=Optimised  visibilities=1032+2^17+2^18+2^19  genFPC=off  floatRounding=correct  advOptions=[]  version=20130821
  Const : DSPBAPrim/Const  primtype=const  nInputs=0  nOutputs=1  omode=Inherit via internal rule  otype=sfix(16)  scale=2^-15  rndmethod=Unbiased  factor=1  satmethod=Symmetric  shift_vec=[0 1 2 -1]  value=0  inPortNames=['+'; '+';]  outPortNames=[' ']  dspbaimage=dspba_prim.jpg  text=fprintf('%s', num2str(value));  style=Optimised  visibilities=8 + 1024  floatPrecision=float32_m23  version=20120820
  Convert1 : DSPBAPrim/Convert  primtype=convert  nInputs=1  nOutputs=1  omode=Specify via dialog  otype=uint(16)  scale=2^-0  rndmethod=Biased  factor=1  satmethod=Asymmetric  shift_vec=[0 1 2 -1]  value=round([0:255]/17)  inPortNames=[' '; ' ';]  outPortNames=[' '; 'c']  dspbaimage=dspba_prim.jpg  text=fprintf('convert');  style=Optimised  visibilities=8+64+256+2^17  clipdetect=off  floatPrecision=float32_m23  advOptions=[]  version=20130211
  Convert2 : DSPBAPrim/Convert  primtype=convert  nInputs=1  nOutputs=1  omode=Specify via dialog  otype=uint(16)  scale=2^-0  rndmethod=Biased  factor=1  satmethod=Asymmetric  shift_vec=[0 1 2 -1]  value=round([0:255]/17)  inPortNames=[' '; ' ';]  outPortNames=[' '; 'c']  dspbaimage=dspba_prim.jpg  text=fprintf('convert');  style=Optimised  visibilities=8+64+256+2^17  clipdetect=off  floatPrecision=float32_m23  advOptions=[]  version=20130211
  Convert3 : DSPBAPrim/Convert  primtype=convert  nInputs=1  nOutputs=1  omode=Specify via dialog  otype=uint(16)  scale=2^-0  rndmethod=Biased  factor=1  satmethod=Asymmetric  shift_vec=[0 1 2 -1]  value=round([0:255]/17)  inPortNames=[' '; ' ';]  outPortNames=[' '; 'c']  dspbaimage=dspba_prim.jpg  text=fprintf('convert');  style=Optimised  visibilities=8+64+256+2^17  clipdetect=off  floatPrecision=float32_m23  advOptions=[]  version=20130211
  MUX3_u : Subsystem
  MUX3_u1 : Subsystem
  MUX3_u2 : Subsystem
  MinMax : DSPBAPrim/MinMax  primtype=minmaxfunc  nInputs=2  nOutputs=1  omode=Inherit via internal rule  otype=sfix(16)  scale=2^-15  rndmethod=Unbiased  factor=1  satmethod=Symmetric  shift_vec=[0 1 2 -1]  value=0  inPortNames=[' '; ' ';]  outPortNames=[' ']  dspbaimage=dspba_prim.jpg  text=disp('min');  style=Optimised  visibilities=8+2^17  functionExpr=sat  advOptions=[]  version=20121130
  MinMax1 : DSPBAPrim/MinMax  primtype=minmaxfunc  nInputs=2  nOutputs=1  omode=Inherit via internal rule  otype=sfix(16)  scale=2^-15  rndmethod=Unbiased  factor=1  satmethod=Symmetric  shift_vec=[0 1 2 -1]  value=0  inPortNames=[' '; ' ';]  outPortNames=[' ']  dspbaimage=dspba_prim.jpg  text=disp('min');  style=Optimised  visibilities=8+2^17  functionExpr=sat  advOptions=[]  version=20121130
  MinMax2 : DSPBAPrim/MinMax  primtype=minmaxfunc  nInputs=2  nOutputs=1  omode=Inherit via internal rule  otype=sfix(16)  scale=2^-15  rndmethod=Unbiased  factor=1  satmethod=Symmetric  shift_vec=[0 1 2 -1]  value=0  inPortNames=[' '; ' ';]  outPortNames=[' ']  dspbaimage=dspba_prim.jpg  text=disp('min');  style=Optimised  visibilities=8+2^17  functionExpr=sat  advOptions=[]  version=20121130
  Negate : DSPBAPrim/Negate  primtype=negate  nInputs=1  nOutputs=1  omode=Inherit via internal rule  otype=sfix(16)  scale=2^-15  rndmethod=Unbiased  factor=1  satmethod=Symmetric  shift_vec=[0 1 2 -1]  value=0  inPortNames=[' '; ' ';]  outPortNames=[' ']  dspbaimage=dspba_prim.jpg  text=fprintf('-x');  style=Optimised  visibilities=8  version=20090407
  Negate3 : DSPBAPrim/Negate  primtype=negate  nInputs=1  nOutputs=1  omode=Inherit via internal rule  otype=sfix(16)  scale=2^-15  rndmethod=Unbiased  factor=1  satmethod=Symmetric  shift_vec=[0 1 2 -1]  value=0  inPortNames=[' '; ' ';]  outPortNames=[' ']  dspbaimage=dspba_prim.jpg  text=fprintf('-x');  style=Optimised  visibilities=8  version=20090407
  Negate4 : DSPBAPrim/Negate  primtype=negate  nInputs=1  nOutputs=1  omode=Inherit via internal rule  otype=sfix(16)  scale=2^-15  rndmethod=Unbiased  factor=1  satmethod=Symmetric  shift_vec=[0 1 2 -1]  value=0  inPortNames=[' '; ' ';]  outPortNames=[' ']  dspbaimage=dspba_prim.jpg  text=fprintf('-x');  style=Optimised  visibilities=8  version=20090407
  ReinterpretCast : DSPBAPrim/ReinterpretCast  primtype=reinterpret  nInputs=1  nOutputs=1  omode=Specify via dialog  otype=uint(16)  scale=2^-1  rndmethod=Unbiased  factor=1  satmethod=Symmetric  shift_vec=[0 1 2 -1]  value=0  inPortNames=[' '; ' ';]  outPortNames=[' ']  dspbaimage=dspba_prim.jpg  text=fprintf('Reinterp\nCast', value);  style=Optimised  visibilities=8  floatPrecision=float32_m23  version=20120601
  Out_u : Outport
  Out_v : Outport  Port=2
  Out_w : Outport  Port=3
  wires:
  Convert3/1 -> MinMax2/1
  Convert2/1 -> MinMax1/1
  Convert1/1 -> MinMax/1
  Add3/1 -> Convert3/1
  Add2/1 -> Convert2/1
  B3p/1 -> MUX3_u2/4(Inp3)
  Negate4/1 -> MUX3_u2/2(Inp1)
  B3m/1 -> MUX3_u1/2(Inp1)
  ReinterpretCast/1 -> Add2/2, Add3/2, Add1/2
  MUX3_u/1(Out13) -> Add1/1
  Max/1 -> ReinterpretCast/1, MinMax/2, MinMax2/2, MinMax1/2
  A/1 -> MUX3_u/3(Inp2)
  Sel/1 -> MUX3_u/1(Sel), MUX3_u1/1(Sel), MUX3_u2/1(Sel)
  Negate/1 -> MUX3_u/4(Inp3)
  Sum/1 -> MUX3_u/2(Inp1), Negate4/1
  D/1 -> MUX3_u1/4(Inp3), Negate/1
  Add1/1 -> Convert1/1
  Negate3/1 -> MUX3_u2/3(Inp2)
  MUX3_u1/1(Out13) -> Add2/1
  MUX3_u2/1(Out13) -> Add3/1
  B/1 -> Negate3/1, MUX3_u1/3(Inp2)
  Const/1 -> MinMax1/3, MinMax2/3, MinMax/3
  MinMax1/1 -> Out_v/1
  MinMax/1 -> Out_u/1
  MinMax2/1 -> Out_w/1

== system foc_blocks/FL_fixp16/SVM/SectorSel ==
  D : Inport
  B : Inport  Port=2
  Sum : Inport  Port=3
  And{,1..4} (5 alike) : DSPBAPrim/And  primtype=and  nInputs=2  nOutputs=1  omode=Inherit via internal rule  otype=sfix(16)  scale=2^-15  rndmethod=Unbiased  factor=1  satmethod=Symmetric  shift_vec=[0 1 2 -1]  value=0  inPortNames=[' '; ' '; ' '; ' '; ' '; ' '; ' '; ' '; ' '; ' '; ' '; ' '; ' '; ' '; ' '; ' '; ]  outPortNames=[' ']  dspbaimage=dspba_prim.jpg  text=fprintf('&');  style=Optimised  visibilities=8+2  version=20090407
  CmpGE : DSPBAPrim/CmpGE  primtype=cmpgte  nInputs=2  nOutputs=1  omode=boolean  otype=sfix(16)  scale=2^-15  rndmethod=Unbiased  factor=1  satmethod=Symmetric  shift_vec=[0 1 2 -1]  value=0  inPortNames=['a'; 'b';]  outPortNames=[' ']  dspbaimage=dspba_prim.jpg  text=fprintf('a>=b');  style=Optimised  visibilities=0  advOptions=[]  version=20130117
  CmpGE1 : DSPBAPrim/CmpGE  primtype=cmpgte  nInputs=2  nOutputs=1  omode=boolean  otype=sfix(16)  scale=2^-15  rndmethod=Unbiased  factor=1  satmethod=Symmetric  shift_vec=[0 1 2 -1]  value=0  inPortNames=['a'; 'b';]  outPortNames=[' ']  dspbaimage=dspba_prim.jpg  text=fprintf('a>=b');  style=Optimised  visibilities=0  advOptions=[]  version=20130117
  CmpGE2 : DSPBAPrim/CmpGE  primtype=cmpgte  nInputs=2  nOutputs=1  omode=boolean  otype=sfix(16)  scale=2^-15  rndmethod=Unbiased  factor=1  satmethod=Symmetric  shift_vec=[0 1 2 -1]  value=0  inPortNames=['a'; 'b';]  outPortNames=[' ']  dspbaimage=dspba_prim.jpg  text=fprintf('a>=b');  style=Optimised  visibilities=0  advOptions=[]  version=20130117
  Const : DSPBAPrim/Const  primtype=const  nInputs=0  nOutputs=1  omode=Inherit via internal rule  otype=sfix(16)  scale=2^-15  rndmethod=Unbiased  factor=1  satmethod=Symmetric  shift_vec=[0 1 2 -1]  value=0  inPortNames=['+'; '+';]  outPortNames=[' ']  dspbaimage=dspba_prim.jpg  text=fprintf('%s', num2str(value));  style=Optimised  visibilities=8 + 1024  floatPrecision=float32_m23  version=20120820
  Const1 : DSPBAPrim/Const  primtype=const  nInputs=0  nOutputs=1  omode=Inherit via internal rule  otype=sfix(16)  scale=2^-15  rndmethod=Unbiased  factor=1  satmethod=Symmetric  shift_vec=[0 1 2 -1]  value=0  inPortNames=['+'; '+';]  outPortNames=[' ']  dspbaimage=dspba_prim.jpg  text=fprintf('%s', num2str(value));  style=Optimised  visibilities=8 + 1024  floatPrecision=float32_m23  version=20120820
  Const2 : DSPBAPrim/Const  primtype=const  nInputs=0  nOutputs=1  omode=Inherit via internal rule  otype=sfix(16)  scale=2^-15  rndmethod=Unbiased  factor=1  satmethod=Symmetric  shift_vec=[0 1 2 -1]  value=1  inPortNames=['+'; '+';]  outPortNames=[' ']  dspbaimage=dspba_prim.jpg  text=fprintf('%s', num2str(value));  style=Optimised  visibilities=8 + 1024  floatPrecision=float32_m23  version=20120820
  Const3 : DSPBAPrim/Const  primtype=const  nInputs=0  nOutputs=1  omode=Inherit via internal rule  otype=sfix(16)  scale=2^-15  rndmethod=Unbiased  factor=1  satmethod=Symmetric  shift_vec=[0 1 2 -1]  value=2  inPortNames=['+'; '+';]  outPortNames=[' ']  dspbaimage=dspba_prim.jpg  text=fprintf('%s', num2str(value));  style=Optimised  visibilities=8 + 1024  floatPrecision=float32_m23  version=20120820
  Const4 : DSPBAPrim/Const  primtype=const  nInputs=0  nOutputs=1  omode=Inherit via internal rule  otype=sfix(16)  scale=2^-15  rndmethod=Unbiased  factor=1  satmethod=Symmetric  shift_vec=[0 1 2 -1]  value=0  inPortNames=['+'; '+';]  outPortNames=[' ']  dspbaimage=dspba_prim.jpg  text=fprintf('%s', num2str(value));  style=Optimised  visibilities=8 + 1024  floatPrecision=float32_m23  version=20120820
  Const5 : DSPBAPrim/Const  primtype=const  nInputs=0  nOutputs=1  omode=Inherit via internal rule  otype=sfix(16)  scale=2^-15  rndmethod=Unbiased  factor=1  satmethod=Symmetric  shift_vec=[0 1 2 -1]  value=1  inPortNames=['+'; '+';]  outPortNames=[' ']  dspbaimage=dspba_prim.jpg  text=fprintf('%s', num2str(value));  style=Optimised  visibilities=8 + 1024  floatPrecision=float32_m23  version=20120820
  Const6 : DSPBAPrim/Const  primtype=const  nInputs=0  nOutputs=1  omode=Inherit via internal rule  otype=sfix(16)  scale=2^-15  rndmethod=Unbiased  factor=1  satmethod=Symmetric  shift_vec=[0 1 2 -1]  value=2  inPortNames=['+'; '+';]  outPortNames=[' ']  dspbaimage=dspba_prim.jpg  text=fprintf('%s', num2str(value));  style=Optimised  visibilities=8 + 1024  floatPrecision=float32_m23  version=20120820
  Mux{1..5} (5 alike) : DSPBAPrim/Mux  primtype=mux  nInputs=evalAionMaskParam(gcb,'value',1)+1  nOutputs=1  omode=Inherit via internal rule  otype=sfix(16)  scale=2^-15  rndmethod=Unbiased  factor=1  satmethod=Symmetric  shift_vec=[0 1 2 -1]  value=2  inPortNames=['s '; 'd0'; 'd1'; 'd2'; 'd3'; 'd4'; 'd5'; 'd6'; 'd7'; 'd8'; 'd9';]  outPortNames=[' ']  dspbaimage=dspba_prim.jpg  text=fprintf('%s', primtype);  style=Optimised  visibilities=1032  version=20131025
  Not : DSPBAPrim/Not  primtype=not  nInputs=1  nOutputs=1  omode=Inherit via internal rule  otype=sfix(16)  scale=2^-15  rndmethod=Unbiased  factor=1  satmethod=Symmetric  shift_vec=[0 1 2 -1]  value=0  inPortNames=[' '; ' ';]  outPortNames=[' ']  dspbaimage=dspba_prim.jpg  text=fprintf('~');  style=Optimised  visibilities=8  version=20090407
  Not1 : DSPBAPrim/Not  primtype=not  nInputs=1  nOutputs=1  omode=Inherit via internal rule  otype=sfix(16)  scale=2^-15  rndmethod=Unbiased  factor=1  satmethod=Symmetric  shift_vec=[0 1 2 -1]  value=0  inPortNames=[' '; ' ';]  outPortNames=[' ']  dspbaimage=dspba_prim.jpg  text=fprintf('~');  style=Optimised  visibilities=8  version=20090407
  Not2 : DSPBAPrim/Not  primtype=not  nInputs=1  nOutputs=1  omode=Inherit via internal rule  otype=sfix(16)  scale=2^-15  rndmethod=Unbiased  factor=1  satmethod=Symmetric  shift_vec=[0 1 2 -1]  value=0  inPortNames=[' '; ' ';]  outPortNames=[' ']  dspbaimage=dspba_prim.jpg  text=fprintf('~');  style=Optimised  visibilities=8  version=20090407
  sel : Outport
  wires:
  Const/1 -> CmpGE2/2, CmpGE1/2, CmpGE/2
  And/1 -> Mux1/1
  Const5/1 -> Mux4/3
  Mux5/1 -> sel/1
  CmpGE/1 -> And/2, Not/1, And2/2
  Not2/1 -> And3/1, And1/2
  And3/1 -> Mux4/1
  And4/1 -> Mux5/1
  Sum/1 -> CmpGE2/1
  CmpGE1/1 -> Not1/1, And1/1
  D/1 -> CmpGE/1
  CmpGE2/1 -> Not2/1, And4/2, And/1
  Const1/1 -> Mux1/2
  Const3/1 -> Mux2/3
  B/1 -> CmpGE1/1
  Mux4/1 -> Mux5/2
  Mux3/1 -> Mux4/2
  Const4/1 -> Mux3/3
  Not1/1 -> And4/1, And2/1
  And2/1 -> Mux3/1
  Mux1/1 -> Mux2/2
  Const6/1 -> Mux5/3
  Mux2/1 -> Mux3/2
  Not/1 -> And3/2
  And1/1 -> Mux2/1
  Const2/1 -> Mux1/3
